simulink library "powerRatio"  (R2018b)
settings: Solver=VariableStepAuto  StartTime=0.0  StopTime=10.0  RelTol=1e-3
libraries: flowSpeedMapping_ul x1, runningAvg_ul x1
settings Model: Creator=MAE-NCSUCORE  LastModifiedBy=mae-ncsucore

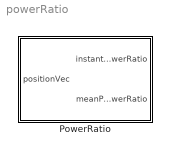
== system powerRatio ==
  PowerRatio : Subsystem  mask{Value=10, Value1=1}
      mask prompts: Value "Water Channel Hz"; Value1 "Reset"
      mask TypeOptions Value: waterChannelHz/Value
      mask TypeOptions Value1: reset/Value

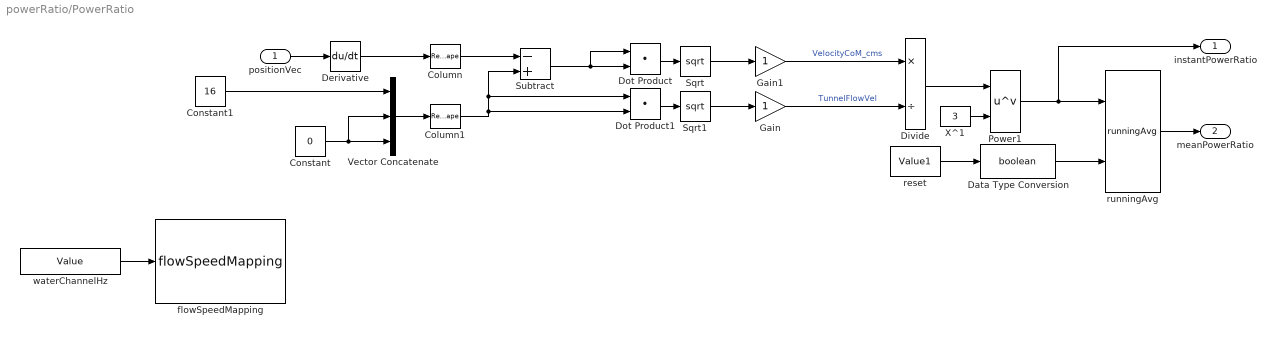
== system powerRatio/PowerRatio ==
  positionVec : Inport
  Column : Reshape  OutputDimensionality=Column vector (2-D)
  Column1 : Reshape  OutputDimensionality=Column vector (2-D)
  Constant : Constant  Value=0
  Constant1 : Constant  Value=16
  Data Type Conversion : DataTypeConversion  OutDataTypeStr=boolean
  Derivative : Derivative
  Divide : Product  Inputs=*/
  Dot Product : DotProduct  InputSameDT=on  OutDataTypeStr=Inherit: Inherit via internal rule
  Dot Product1 : DotProduct  InputSameDT=on  OutDataTypeStr=Inherit: Inherit via internal rule
  Gain : Gain
  Gain1 : Gain
  Power1 : Math  Operator=pow  SaturateOnIntegerOverflow=on
  Sqrt : Sqrt  SaturateOnIntegerOverflow=on
  Sqrt1 : Sqrt  SaturateOnIntegerOverflow=on
  Subtract : Sum  Inputs=-+
  Vector Concatenate : Concatenate  NumInputs=3
  X^1 : Constant  Value=3
  flowSpeedMapping : flowSpeedMapping_ul/flowSpeedMapping  Value=-0.00934  Gain=0.017
  reset : Constant  Value=Value1
  runningAvg : runningAvg_ul/runningAvg  SystemSampleTime=-1
  waterChannelHz : Constant  Value=Value
  instantPowerRatio : Outport
  meanPowerRatio : Outport  Port=2
  wires:
  X^1/1 -> Power1/2
  Vector Concatenate/1 -> Column1/1
  Column/1 -> Subtract/1
  Derivative/1 -> Column/1
  positionVec/1 -> Derivative/1
  Sqrt/1 -> Gain1/1
  Divide/1 -> Power1/1
  Power1/1 -> instantPowerRatio/1, runningAvg/1
  Dot Product/1 -> Sqrt/1
  Subtract/1 -> Dot Product/2, Dot Product/1
  Constant/1 -> Vector Concatenate/2, Vector Concatenate/3
  runningAvg/1 -> meanPowerRatio/1
  waterChannelHz/1 -> flowSpeedMapping/1
  reset/1 -> Data Type Conversion/1
  Column1/1 -> Dot Product1/2, Dot Product1/1, Subtract/2
  Dot Product1/1 -> Sqrt1/1
  Sqrt1/1 -> Gain/1
  Data Type Conversion/1 -> runningAvg/2
  Constant1/1 -> Vector Concatenate/1
  Gain/1 -> Divide/2  "TunnelFlowVel"
  Gain1/1 -> Divide/1  "VelocityCoM_cms"
